simulink model "Unit_Delay"  (R2023b)
settings: Solver=FixedStepAuto  StartTime=0.0  StopTime=10.0  FixedStep=0.5  RelTol=1e-3
settings Model: Creator=hp  LastModifiedBy=hp

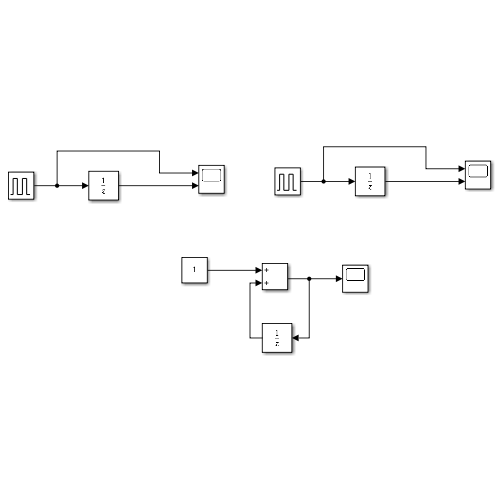
[thumbnail: Simulink's stored preview of the top-level diagram]
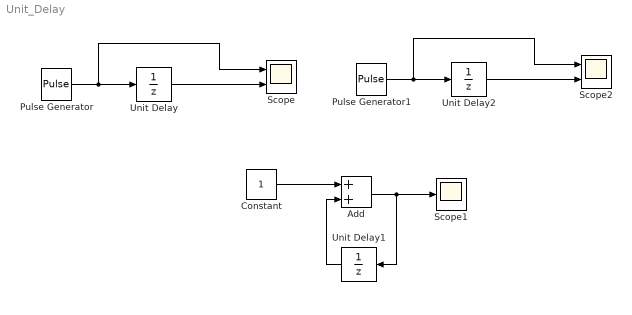
== system Unit_Delay ==
  Add : Sum
  Constant : Constant
  Pulse Generator : DiscretePulseGenerator  PulseType=Time based  Period=10  PulseWidth=25
  Pulse Generator1 : DiscretePulseGenerator  PulseType=Time based  Period=10  PulseWidth=50
  Scope : Scope  NumInputPorts=2
  Scope1 : Scope
  Scope2 : Scope  NumInputPorts=2
  Unit Delay : UnitDelay  SampleTime=0.2  HasFrameUpgradeWarning=on
  Unit Delay1 : UnitDelay  HasFrameUpgradeWarning=on
  Unit Delay2 : UnitDelay  SampleTime=-1  HasFrameUpgradeWarning=on
  wires:
  Pulse Generator/1 -> Scope/1, Unit Delay/1
  Unit Delay/1 -> Scope/2
  Constant/1 -> Add/1
  Add/1 -> Unit Delay1/1, Scope1/1
  Unit Delay1/1 -> Add/2
  Unit Delay2/1 -> Scope2/2
  Pulse Generator1/1 -> Unit Delay2/1, Scope2/1
